simulink model "debugECDD"  (Simulink 7.2)
settings: Solver=ode1  StartTime=0.0  StopTime=50  FixedStep=0.002  RelTol=1e-3
values from neighbouring files (symbols this model uses):
  a = param.a    [DSC_Control_Analysis.m]    (also in DSC_Control_Analysis_Exp.m; DSC_Speed_Control_Analysis.m; EmpiricalTireCurves.m = 1.35; FFW_Fx.m = sqrt(curvature/(2*clothoidLength)))
  b = 1.15    [EmpiricalTireCurves.m]
  Cfls = Cfl    [EC_params_nissan.m]
  Crls = Crl    [EC_params_nissan.m]
  Iz = param.Iz    [DSC_Control_Analysis.m]    (also in DSC_Control_Analysis_Exp.m; DSC_Speed_Control_Analysis.m; EmpiricalTireCurves.m = 1300)
  K = 10    [EC_params_nissan.m]
  Ks = -10    [EC_params_nissan.m]
  Ksl = -10    [EC_params_nissan.m]
  Kt = 40000    [EC_params_nissan.m]
  Ku = -40000    [EC_params_nissan.m]
  m = 1724    [EmpiricalTireCurves.m]
  mu_s = mu_p    (= 0.6)    [EC_params_nissan.m]    (also in EmpiricalTireCurves.m = 0.55)
  Ns = 10    [EC_params_nissan.m]
  q = 1    [EC_params_nissan.m]
undefined symbols (not defined in the file or in its folder): c, Cfl, Crl, dden, denafilt, dnum, filtera, filterb, h_roll, Ifalphaparam, numafilt, param, rfl, rfr, rrl, rrr, sglu, slimFxl, slimFxu, sliml, slimMll, slimMlr, slimMul, slimMur, slimu, steering_limit, tw_m, wc
libraries: simulink x15, xpclib x3, UserBlocks x1
(part 2 of 3)

== system debugECDD/Envelope control with Differential drive/envelope controller with DD/control_on ==
  note: [Control on condition]
      | - Switch ON
      | - Brake OFF
      | - Vx > 2m/s
      | - GPS works
  Fault switch : Inport  OutDataType=sfix(16)  OutScaling=2^0
  brake_sw : Inport  Port=2  OutDataType=sfix(16)  OutScaling=2^0
  Vx : Inport  Port=3  OutDataType=sfix(16)  OutScaling=2^0
  Bus Selector1 : BusSelector  OutputSignals=signal2.Velocity Solution Status,signal1.Attitude Status
  Constant : Constant  Value=2  OutDataType=sfix(16)  OutScaling=2^0
  Constant1 : Constant  Value=3  OutDataType=sfix(16)  OutScaling=2^0
  Constant2 : Constant  Value=4  OutDataType=sfix(16)  OutScaling=2^0
  Data Type Conversion1 : DataTypeConversion  OutDataTypeMode=double  OutDataType=sfix(16)  OutScaling=2^0  OutDataTypeStr=double  RndMeth=Nearest  SaturateOnIntegerOverflow=on
  Data Type Conversion2 : DataTypeConversion  OutDataTypeMode=double  OutDataType=sfix(16)  OutScaling=2^0  OutDataTypeStr=double  RndMeth=Nearest  SaturateOnIntegerOverflow=on
  Data Type Conversion3 : DataTypeConversion  OutDataType=sfix(16)  OutScaling=2^0  RndMeth=Nearest  SaturateOnIntegerOverflow=on
  Logical Operator : Logic  Operator=NOT  AllPortsSameDT=off  OutDataTypeMode=boolean  OutDataTypeStr=boolean
  Logical Operator{1..4} (4 alike) : Logic  AllPortsSameDT=off  OutDataTypeMode=boolean  OutDataTypeStr=boolean
  Relational Operator : RelationalOperator  Operator=>  LogicOutDataTypeMode=boolean  OutDataTypeStr=boolean
  Relational Operator1 : RelationalOperator  Operator===  LogicOutDataTypeMode=boolean  OutDataTypeStr=boolean
  Relational Operator2 : RelationalOperator  Operator===  LogicOutDataTypeMode=boolean  OutDataTypeStr=boolean
  Rounding Function : Rounding  Operator=round
  Rounding Function1 : Rounding  Operator=round
  ON FLAG : Outport  OutDataType=sfix(16)  OutScaling=2^0
  tag scope: ECDDbrake=global, ECDDspeed=global, GPS_condition=global
  wires:
  Data Type Conversion3/1 -> [ECDDbrake], Logical Operator/1
  Logical Operator4/1 -> ON FLAG/1
  Logical Operator3/1 -> Logical Operator4/2, [GPS_condition]
  Logical Operator2/1 -> Logical Operator4/1
  Relational Operator2/1 -> Logical Operator3/2
  Relational Operator1/1 -> Logical Operator3/1
  Constant2/1 -> Relational Operator2/2
  Rounding Function1/1 -> Relational Operator2/1
  Constant1/1 -> Relational Operator1/1
  Rounding Function/1 -> Relational Operator1/2
  Data Type Conversion1/1 -> Rounding Function1/1
  Data Type Conversion2/1 -> Rounding Function/1
  [global_GPS] -> Bus Selector1/1
  Bus Selector1/2 -> Data Type Conversion1/1  "<Attitude Status>"
  Bus Selector1/1 -> Data Type Conversion2/1  "<Velocity Solution Status>"
  Relational Operator/1 -> [ECDDspeed], Logical Operator2/2
  Logical Operator1/1 -> Logical Operator2/1
  Constant/1 -> Relational Operator/2
  Vx/1 -> Relational Operator/1
  Logical Operator/1 -> Logical Operator1/2
  Fault switch/1 -> Logical Operator1/1
  brake_sw/1 -> Data Type Conversion3/1

== system debugECDD/Envelope control with Differential drive/envelope controller with DD/drive_dynamics ==
  In1 : Inport  OutDataType=sfix(16)  OutScaling=2^0
  Demux : Demux
  Discrete Transfer Fcn{,1..3} (4 alike) : DiscreteTransferFcn  Numerator=0.3297  Denominator=[1 -0.6703]  SampleTime=0.002
  Mux : Mux
  Out1 : Outport  OutDataType=sfix(16)  OutScaling=2^0
  wires:
  In1/1 -> Demux/1
  Mux/1 -> Out1/1
  Demux/1 -> Discrete Transfer Fcn/1
  Demux/2 -> Discrete Transfer Fcn1/1
  Demux/3 -> Discrete Transfer Fcn2/1
  Demux/4 -> Discrete Transfer Fcn3/1
  Discrete Transfer Fcn/1 -> Mux/1
  Discrete Transfer Fcn1/1 -> Mux/2
  Discrete Transfer Fcn2/1 -> Mux/3
  Discrete Transfer Fcn3/1 -> Mux/4

== system debugECDD/Envelope control with Differential drive/envelope controller with DD/reaction force control ==
  reaction 1 : Inport  OutDataType=sfix(16)  OutScaling=2^0
  reaction 2 : Inport  Port=2  OutDataType=sfix(16)  OutScaling=2^0
  Constant : Constant  Value=0  OutDataType=sfix(16)  OutScaling=2^0
  Constant1 : Constant  Value=0  OutDataType=sfix(16)  OutScaling=2^0
  Constant2 : Constant  Value=0  OutDataType=sfix(16)  OutScaling=2^0
  Terminator : Terminator
  Terminator1 : Terminator
  steer force : Outport  OutDataType=sfix(16)  OutScaling=2^0
  ACC pedal force : Outport  Port=2  OutDataType=sfix(16)  OutScaling=2^0
  Brake pedal force1 : Outport  Port=3  OutDataType=sfix(16)  OutScaling=2^0
  wires:
  reaction 2/1 -> Terminator1/1
  reaction 1/1 -> Terminator/1
  Constant2/1 -> Brake pedal force1/1
  Constant1/1 -> ACC pedal force/1
  Constant/1 -> steer force/1

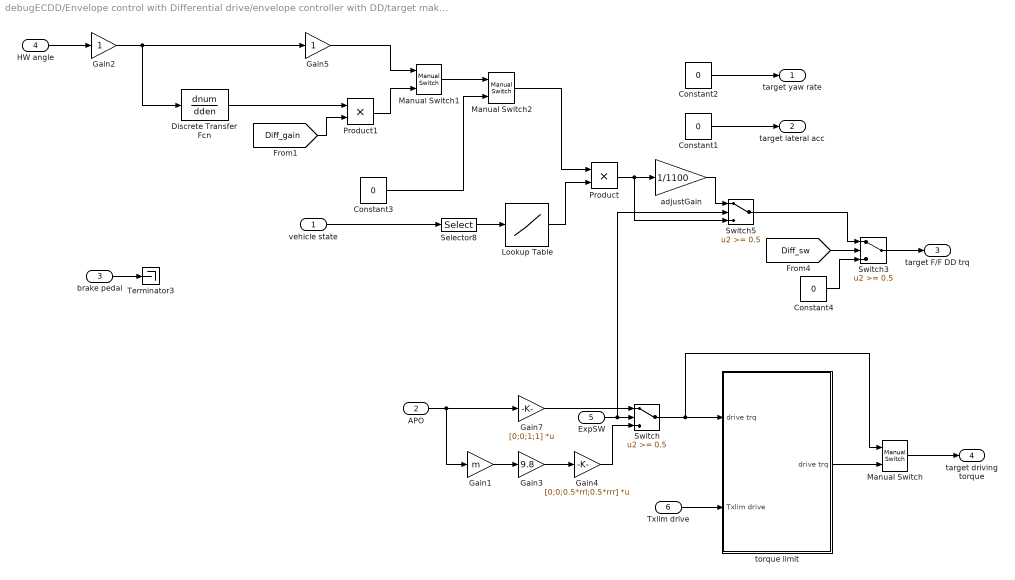
== system debugECDD/Envelope control with Differential drive/envelope controller with DD/target making ==
  vehicle state : Inport  OutDataType=sfix(16)  OutScaling=2^0
  APO : Inport  Port=2  OutDataType=sfix(16)  OutScaling=2^0
  brake pedal : Inport  Port=3  OutDataType=sfix(16)  OutScaling=2^0
  HW angle : Inport  Port=4  OutDataType=sfix(16)  OutScaling=2^0
  ExpSW : Inport  Port=5  OutDataType=sfix(16)  OutScaling=2^0
  Txlim drive : Inport  Port=6  OutDataType=sfix(16)  OutScaling=2^0
  Constant{1..4} (4 alike) : Constant  Value=0  OutDataType=sfix(16)  OutScaling=2^0
  Discrete Transfer Fcn : DiscreteTransferFcn  Numerator=dnum  Denominator=dden  SampleTime=0.002
  Gain1 : Gain  Gain=m  ParameterDataType=sfix(16)  ParameterScaling=2^0  OutDataType=sfix(16)  OutScaling=2^0
  Gain2 : Gain  ParameterDataType=sfix(16)  ParameterScaling=2^0  OutDataType=sfix(16)  OutScaling=2^0
  Gain3 : Gain  Gain=9.8  ParameterDataType=sfix(16)  ParameterScaling=2^0  OutDataType=sfix(16)  OutScaling=2^0
  Gain4 : Gain  Gain=[0;0;0.5*rrl;0.5*rrr]  Multiplication=Matrix(K*u)  ParameterDataType=sfix(16)  ParameterScaling=2^0  OutDataType=sfix(16)  OutScaling=2^0
  Gain5 : Gain  ParameterDataType=sfix(16)  ParameterScaling=2^0  OutDataType=sfix(16)  OutScaling=2^0
  Gain7 : Gain  Gain=[0;0;1;1]  Multiplication=Matrix(K*u)  ParameterDataType=sfix(16)  ParameterScaling=2^0  OutDataType=sfix(16)  OutScaling=2^0
  Lookup Table : Lookup  InputValues=[0;1;2;3]  Table=[0;0;1;1]  OutDataType=sfix(16)  OutScaling=2^0
  Manual Switch : simulink/Signal Routing/Manual Switch  SystemSampleTime=-1  sw=0  action=0  varsize=off
  Manual Switch1 : simulink/Signal Routing/Manual Switch  SystemSampleTime=-1  sw=0  action=0  varsize=off
  Manual Switch2 : simulink/Signal Routing/Manual Switch  SystemSampleTime=-1  sw=1  action=0  varsize=off
  Product : Product  OutDataType=sfix(16)  OutScaling=2^0  RndMeth=Zero
  Product1 : Product  OutDataType=sfix(16)  OutScaling=2^0  RndMeth=Zero
  Selector8 : Selector  InputPortWidth=12  IndexOptions=Index vector (dialog)  Indices=5  OutputSizes=1
  Switch : Switch  Threshold=0.5  OutDataType=sfix(16)  OutScaling=2^0
  Switch3 : Switch  Threshold=0.5
  Switch5 : Switch  Threshold=0.5
  Terminator3 : Terminator
  adjustGain : Gain  Gain=1/1100  ParameterDataType=sfix(16)  ParameterScaling=2^0  OutDataType=sfix(16)  OutScaling=2^0
  torque limit : Subsystem
  target yaw rate : Outport  OutDataType=sfix(16)  OutScaling=2^0
  target lateral acc : Outport  Port=2  OutDataType=sfix(16)  OutScaling=2^0
  target F/F DD trq : Outport  Port=3  OutDataType=sfix(16)  OutScaling=2^0
  target driving torque : Outport  Port=4  OutDataType=sfix(16)  OutScaling=2^0
  wires:
  Gain3/1 -> Gain4/1
  Gain1/1 -> Gain3/1
  Constant1/1 -> target lateral acc/1
  brake pedal/1 -> Terminator3/1
  ExpSW/1 -> Switch/2, Switch5/2
  Gain4/1 -> Switch/3
  APO/1 -> Gain1/1, Gain7/1
  Gain7/1 -> Switch/1
  Switch/1 -> torque limit/1("drive trq "), Manual Switch/1
  Txlim drive/1 -> torque limit/2(Txlim drive)
  torque limit/1(drive trq) -> Manual Switch/2
  Manual Switch/1 -> target driving torque/1
  Constant2/1 -> target yaw rate/1
  HW angle/1 -> Gain2/1
  Gain2/1 -> Gain5/1, Discrete Transfer Fcn/1
  vehicle state/1 -> Selector8/1
  Selector8/1 -> Lookup Table/1
  Lookup Table/1 -> Product/2
  Product1/1 -> Manual Switch1/2
  Gain5/1 -> Manual Switch1/1
  Manual Switch2/1 -> Product/1
  Manual Switch1/1 -> Manual Switch2/1
  Constant3/1 -> Manual Switch2/2
  [Diff_sw] -> Switch3/2
  Constant4/1 -> Switch3/3
  Switch3/1 -> target F/F DD trq/1
  Discrete Transfer Fcn/1 -> Product1/1
  [Diff_gain] -> Product1/2
  adjustGain/1 -> Switch5/1
  Product/1 -> adjustGain/1, Switch5/3
  Switch5/1 -> Switch3/1

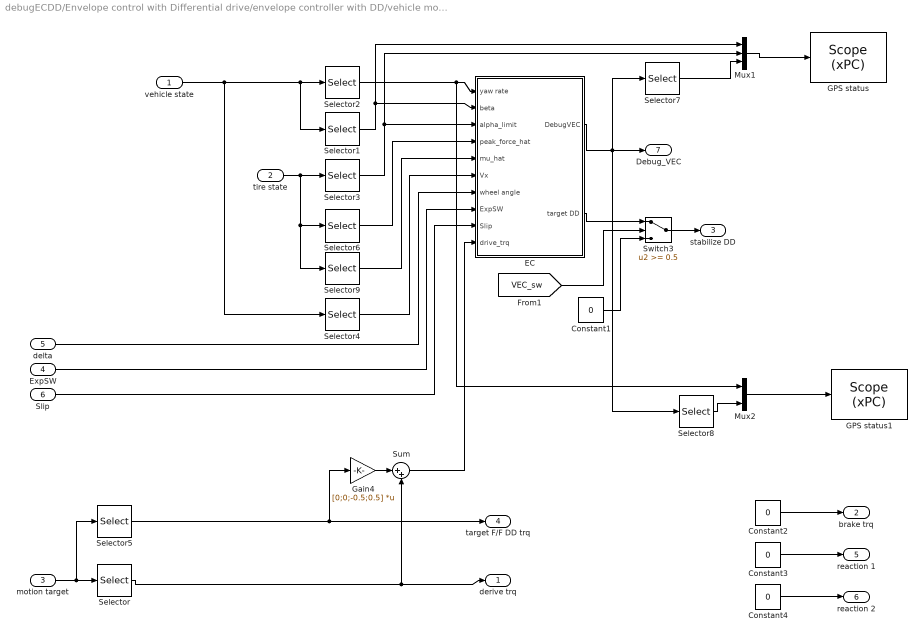
== system debugECDD/Envelope control with Differential drive/envelope controller with DD/vehicle motion control ==
  vehicle state : Inport  OutDataType=sfix(16)  OutScaling=2^0
  tire state : Inport  Port=2  OutDataType=sfix(16)  OutScaling=2^0
  motion target : Inport  Port=3  OutDataType=sfix(16)  OutScaling=2^0
  ExpSW : Inport  Port=4  OutDataType=sfix(16)  OutScaling=2^0
  delta : Inport  Port=5  OutDataType=sfix(16)  OutScaling=2^0
  Slip : Inport  Port=6  OutDataType=sfix(16)  OutScaling=2^0
  Constant{1..4} (4 alike) : Constant  Value=0  OutDataType=sfix(16)  OutScaling=2^0
  EC : Subsystem
  GPS status : xpclib/Misc./Scope (xPC)   SystemSampleTime=-1  scopeno=1  scopetype=Target  autostart=on  viewmode=Graphical sliding  formatstr='%15.6f'  grid=on  ylimits=[-1,1]  nosamples=round(1/Ts)  noprepostsamples=0  interleave=1  triggermode=FreeRun  triggersignal=1  triggerlevel=0.0  triggerslope=Either  triggerscope=1  triggersample=0  filename=data.dat  mode=Lazy  writesize=512  autorestart=off
  GPS status1 : xpclib/Misc./Scope (xPC)   SystemSampleTime=-1  scopeno=4  scopetype=Target  autostart=on  viewmode=Graphical sliding  formatstr='%15.6f'  grid=on  ylimits=[-1,1]  nosamples=round(1/Ts)  noprepostsamples=0  interleave=1  triggermode=FreeRun  triggersignal=1  triggerlevel=0.0  triggerslope=Either  triggerscope=1  triggersample=0  filename=data.dat  mode=Lazy  writesize=512  autorestart=off
  Gain4 : Gain  Gain=[0;0;-0.5;0.5]  Multiplication=Matrix(K*u)  ParameterDataType=sfix(16)  ParameterScaling=2^0  OutDataType=sfix(16)  OutScaling=2^0
  Mux1 : Mux  Inputs=3
  Mux2 : Mux  Inputs=2
  Selector : Selector  InputPortWidth=7  IndexOptions=Index vector (dialog)  Indices=[4:7]  OutputSizes=1
  Selector1 : Selector  InputPortWidth=12  IndexOptions=Index vector (dialog)  Indices=12  OutputSizes=1
  Selector2 : Selector  InputPortWidth=12  IndexOptions=Index vector (dialog)  Indices=7  OutputSizes=1
  Selector3 : Selector  InputPortWidth=9  IndexOptions=Index vector (dialog)  Indices=[7:8]  OutputSizes=1
  Selector4 : Selector  InputPortWidth=12  IndexOptions=Index vector (dialog)  Indices=5  OutputSizes=1
  Selector5 : Selector  InputPortWidth=7  IndexOptions=Index vector (dialog)  Indices=3  OutputSizes=1
  Selector6 : Selector  InputPortWidth=9  IndexOptions=Index vector (dialog)  Indices=[3:6]  OutputSizes=1
  Selector7 : Selector  InputPortWidth=11  IndexOptions=Index vector (dialog)  Indices=[8 9]  OutputSizes=1
  Selector8 : Selector  InputPortWidth=11  IndexOptions=Index vector (dialog)  Indices=[6 7]  OutputSizes=1
  Selector9 : Selector  InputPortWidth=9  IndexOptions=Index vector (dialog)  Indices=9  OutputSizes=1
  Sum : Sum  Inputs=|++  OutDataType=sfix(16)  OutScaling=2^0
  Switch3 : Switch  Threshold=0.5
  derive trq : Outport  OutDataType=sfix(16)  OutScaling=2^0
  brake trq : Outport  Port=2  OutDataType=sfix(16)  OutScaling=2^0
  stabilize DD : Outport  Port=3  OutDataType=sfix(16)  OutScaling=2^0
  target F/F DD trq : Outport  Port=4  OutDataType=sfix(16)  OutScaling=2^0
  reaction 1 : Outport  Port=5  OutDataType=sfix(16)  OutScaling=2^0
  reaction 2 : Outport  Port=6  OutDataType=sfix(16)  OutScaling=2^0
  Debug_VEC : Outport  Port=7  OutDataType=sfix(16)  OutScaling=2^0
  wires:
  Mux1/1 -> GPS status/1
  Selector7/1 -> Mux1/3
  EC/1(DebugVEC) -> Selector7/1, Debug_VEC/1, Selector8/1
  Selector4/1 -> EC/6(Vx)
  Constant1/1 -> Switch3/3
  EC/2(target DD) -> Switch3/1
  [VEC_sw] -> Switch3/2
  delta/1 -> EC/7(wheel angle)
  tire state/1 -> Selector3/1, Selector6/1, Selector9/1
  Selector3/1 -> EC/3(alpha_limit), Mux1/2
  Selector1/1 -> Mux1/1, EC/2(beta)
  vehicle state/1 -> Selector1/1, Selector2/1, Selector4/1
  Selector2/1 -> EC/1(yaw rate), Mux2/1
  motion target/1 -> Selector/1, Selector5/1
  Constant4/1 -> reaction 2/1
  Constant3/1 -> reaction 1/1
  Constant2/1 -> brake trq/1
  Mux2/1 -> GPS status1/1
  Selector8/1 -> Mux2/2
  Selector6/1 -> EC/4(peak_force_hat)
  ExpSW/1 -> EC/8(ExpSW)
  Slip/1 -> EC/9(Slip)
  Switch3/1 -> stabilize DD/1
  Selector9/1 -> EC/5(mu_hat)
  Selector/1 -> derive trq/1, Sum/2
  Selector5/1 -> target F/F DD trq/1, Gain4/1
  Gain4/1 -> Sum/1
  Sum/1 -> EC/10(drive_trq)

== system debugECDD/Envelope control with Differential drive/envelope controller with DD/Control switch/Delay ==
  In1 : Inport  OutDataType=sfix(16)  OutScaling=2^0
  Unit Delay{,1..4} (5 alike) : UnitDelay  X0=2  SampleTime=0.002
  Out1 : Outport  OutDataType=sfix(16)  OutScaling=2^0
  wires:
  In1/1 -> Unit Delay/1
  Unit Delay/1 -> Unit Delay1/1
  Unit Delay1/1 -> Unit Delay2/1
  Unit Delay2/1 -> Unit Delay3/1
  Unit Delay3/1 -> Unit Delay4/1
  Unit Delay4/1 -> Out1/1

== system debugECDD/Envelope control with Differential drive/envelope controller with DD/Control switch/Triggered Subsystem1 ==
  In1 : Inport  OutDataType=sfix(16)  OutScaling=2^0
  Trigger : TriggerPort
  Constant : Constant  OutDataType=sfix(16)  OutScaling=2^0
  Constant1 : Constant  OutDataType=sfix(16)  OutScaling=2^0
  Sum : Sum  Inputs=|++  OutDataType=sfix(16)  OutScaling=2^0
  Switch : Switch  Threshold=4.5  OutDataType=sfix(16)  OutScaling=2^0
  Out1 : Outport  OutDataType=sfix(16)  OutScaling=2^0  InitialOutput=2
  wires:
  In1/1 -> Sum/1
  Constant/1 -> Sum/2
  Sum/1 -> Switch/2, Switch/3
  Constant1/1 -> Switch/1
  Switch/1 -> Out1/1

== system debugECDD/Envelope control with Differential drive/envelope controller with DD/Tire force control/limit_cal ==
  muFz : Inport  OutDataType=sfix(16)  OutScaling=2^0
  alpha : Inport  Port=2  OutDataType=sfix(16)  OutScaling=2^0
  ExpSW : Inport  Port=3  OutDataType=sfix(16)  OutScaling=2^0
  stabilize DD : Inport  Port=4  OutDataType=sfix(16)  OutScaling=2^0
  Fx_limit_cal : Subsystem
  Fx_limit_cal1 : Subsystem
  MinMax{1..4} (4 alike) : MinMax  Inputs=2  OutDataType=sfix(16)  OutScaling=2^0
  Mux1 : Mux
  Mux7 : Mux
  RL & RR max : Constant  Value=3  OutDataType=sfix(16)  OutScaling=2^0
  RL & RR max1 : Constant  Value=3  OutDataType=sfix(16)  OutScaling=2^0
  RL min : Constant  Value=0.75  OutDataType=sfix(16)  OutScaling=2^0
  RL min1 : Constant  Value=0.75  OutDataType=sfix(16)  OutScaling=2^0
  RR min : Constant  Value=0.75  OutDataType=sfix(16)  OutScaling=2^0
  RR min1 : Constant  Value=0.75  OutDataType=sfix(16)  OutScaling=2^0
  Selector1 : Selector  InputPortWidth=4  IndexOptions=Index vector (dialog)  Indices=3  OutputSizes=1
  Selector2 : Selector  InputPortWidth=4  IndexOptions=Index vector (dialog)  Indices=3  OutputSizes=1
  Selector3 : Selector  InputPortWidth=4  IndexOptions=Index vector (dialog)  Indices=1  OutputSizes=1
  Selector8 : Selector  InputPortWidth=4  IndexOptions=Index vector (dialog)  Indices=1  OutputSizes=1
  Sum : Sum  Inputs=|++  OutDataType=sfix(16)  OutScaling=2^0
  Sum1 : Sum  Inputs=|++  OutDataType=sfix(16)  OutScaling=2^0
  Switch1 : Switch  Threshold=0.5
  Switch4 : Switch  Threshold=0.5
  adjustGain : Gain  Gain=1/1100  ParameterDataType=sfix(16)  ParameterScaling=2^0  OutDataType=sfix(16)  OutScaling=2^0
  adjustGain1 : Gain  Gain=1/1100  ParameterDataType=sfix(16)  ParameterScaling=2^0  OutDataType=sfix(16)  OutScaling=2^0
  pedal offset : Constant  Value=1.75  OutDataType=sfix(16)  OutScaling=2^0
  pedal offset1 : Constant  Value=1.75  OutDataType=sfix(16)  OutScaling=2^0
  slip_limit_cal1 : Subsystem
  slim : Outport  OutDataType=sfix(16)  OutScaling=2^0
  Txlim : Outport  Port=2  OutDataType=sfix(16)  OutScaling=2^0
  Txlim drive : Outport  Port=3  OutDataType=sfix(16)  OutScaling=2^0
  wires:
  Switch4/1 -> Txlim/1
  Fx_limit_cal/1(Txlim) -> Switch4/3, adjustGain/1
  ExpSW/1 -> Switch4/2, Switch1/2
  slip_limit_cal1/1(slim) -> Fx_limit_cal/2(slim), slim/1
  muFz/1 -> slip_limit_cal1/3(muFz), Fx_limit_cal/3(muFz), Fx_limit_cal1/3(muFz)
  alpha/1 -> slip_limit_cal1/1(alpha), Fx_limit_cal/1(alpha), Fx_limit_cal1/1(alpha)
  Selector8/1 -> MinMax4/1
  Selector1/1 -> MinMax1/1
  RL & RR max/1 -> MinMax4/2, MinMax1/2
  MinMax4/1 -> Mux7/1
  RL min/1 -> Mux7/2
  MinMax1/1 -> Mux7/3
  RR min/1 -> Mux7/4
  Mux7/1 -> Switch4/1
  Sum/1 -> Selector8/1, Selector1/1
  adjustGain/1 -> Sum/1
  pedal offset/1 -> Sum/2
  stabilize DD/1 -> slip_limit_cal1/2(stabilize DD), Fx_limit_cal/4(stabilize DD)
  Switch1/1 -> Txlim drive/1
  Fx_limit_cal1/1(Txlim drive) -> adjustGain1/1, Switch1/3, Fx_limit_cal/5(Txlim drive)
  Selector3/1 -> MinMax3/1
  Selector2/1 -> MinMax2/1
  RL & RR max1/1 -> MinMax2/2, MinMax3/2
  MinMax3/1 -> Mux1/1
  RL min1/1 -> Mux1/2
  MinMax2/1 -> Mux1/3
  RR min1/1 -> Mux1/4
  Mux1/1 -> Switch1/1
  Sum1/1 -> Selector2/1, Selector3/1
  adjustGain1/1 -> Sum1/1
  pedal offset1/1 -> Sum1/2
  slip_limit_cal1/2(slim drive) -> Fx_limit_cal1/2(slim drive)

== system debugECDD/Envelope control with Differential drive/envelope controller with DD/Tire force control/s_cal  ==
  note: Vx
  Omega : Inport  OutDataType=sfix(16)  OutScaling=2^0
  Vx : Inport  Port=2  OutDataType=sfix(16)  OutScaling=2^0
  yaw rate : Inport  Port=3  OutDataType=sfix(16)  OutScaling=2^0
  ExpSW : Inport  Port=4  OutDataType=sfix(16)  OutScaling=2^0
  Add4 : Sum  Inputs=+-  OutDataType=sfix(16)  OutScaling=2^-10
  Add5 : Sum  Inputs=+-  OutDataType=sfix(16)  OutScaling=2^-10
  Butterworth Filter : DiscreteFilter  Numerator=filterb  Denominator=filtera  SampleTime=0.002
  Butterworth Filter1 : DiscreteFilter  Numerator=filterb  Denominator=filtera  SampleTime=0.002
  Demux4 : Demux
  Divide : Product  Inputs=*/  OutDataType=sfix(16)  OutScaling=2^-10
  Divide1 : Product  Inputs=*/  OutDataType=sfix(16)  OutScaling=2^-10
  Gain1 : Gain  Gain=rrl  ParameterDataType=sfix(16)  ParameterScaling=2^0  OutDataType=sfix(16)  OutScaling=2^0
  Gain2 : Gain  Gain=rrr  ParameterDataType=sfix(16)  ParameterScaling=2^0  OutDataType=sfix(16)  OutScaling=2^0
  Gain3 : Gain  Gain=c  ParameterDataType=sfix(16)  ParameterScaling=2^0  OutDataType=sfix(16)  OutScaling=2^0
  Manual Switch : simulink/Signal Routing/Manual Switch  SystemSampleTime=-1  sw=0  action=0  varsize=off
  Manual Switch1 : simulink/Signal Routing/Manual Switch  SystemSampleTime=-1  sw=0  action=0  varsize=off
  Mux : Mux  Inputs=2
  Product : Product  OutDataType=sfix(16)  OutScaling=2^0  RndMeth=Zero
  Relational Operator : RelationalOperator  Operator=<  LogicOutDataTypeMode=boolean  OutDataTypeStr=boolean
  Relational Operator1 : RelationalOperator  Operator=<  LogicOutDataTypeMode=boolean  OutDataTypeStr=boolean
  Saturation : Saturate  UpperLimit=0.99  LowerLimit=-0.99
  Saturation1 : Saturate  UpperLimit=0.99  LowerLimit=-0.99
  Sum : Sum  Inputs=|+-  OutDataType=sfix(16)  OutScaling=2^0
  Sum1 : Sum  Inputs=++|  OutDataType=sfix(16)  OutScaling=2^0
  Switch : Switch  Threshold=0.5
  Switch1 : Switch  Threshold=0.5
  Terminator1 : Terminator
  Terminator2 : Terminator
  prevent zero : Subsystem
  prevent zero1 : Subsystem
  s : Outport  OutDataType=sfix(16)  OutScaling=2^0
  wires:
  Manual Switch1/1 -> Sum1/2, Sum/1
  Gain2/1 -> Relational Operator/2, Add5/2, Switch/1
  Gain1/1 -> Relational Operator1/2, Add4/2, Switch1/1
  Gain3/1 -> Sum1/1, Sum/2
  Sum1/1 -> Relational Operator/1, Add5/1, Switch/3
  Sum/1 -> Relational Operator1/1, Add4/1, Switch1/3
  Product/1 -> Gain3/1
  ExpSW/1 -> Product/2
  yaw rate/1 -> Butterworth Filter1/1, Manual Switch/1
  Demux4/2 -> Terminator1/1
  Demux4/1 -> Terminator2/1
  Mux/1 -> s/1
  Divide1/1 -> Saturation/1
  Divide/1 -> Saturation1/1
  Omega/1 -> Demux4/1
  Add5/1 -> Divide1/1
  Add4/1 -> Divide/1
  Demux4/4 -> Gain2/1
  Demux4/3 -> Gain1/1
  Vx/1 -> Butterworth Filter/1, Manual Switch1/1
  prevent zero/1(Out1) -> Divide/2
  prevent zero1/1(Out1) -> Divide1/2
  Switch/1 -> prevent zero1/1(In1)
  Relational Operator/1 -> Switch/2
  Switch1/1 -> prevent zero/1(In1)
  Relational Operator1/1 -> Switch1/2
  Saturation/1 -> Mux/2
  Saturation1/1 -> Mux/1
  Manual Switch/1 -> Product/1
  Butterworth Filter1/1 -> Manual Switch/2
  Butterworth Filter/1 -> Manual Switch1/2

== system debugECDD/Envelope control with Differential drive/envelope controller with DD/Tire force control/slip_limit ==
  s : Inport  OutDataType=sfix(16)  OutScaling=2^0
  slim : Inport  Port=2  OutDataType=sfix(16)  OutScaling=2^0
  Constant4 : Constant  Value=[0;0]  OutDataType=sfix(16)  OutScaling=2^0
  Data Type Conversion : DataTypeConversion  OutDataType=sfix(16)  OutScaling=2^0
  Data Type Conversion1 : DataTypeConversion  OutDataType=sfix(16)  OutScaling=2^0
  Demux2 : Demux  Outputs=2
  Demux3 : Demux  Outputs=2
  Demux4 : Demux  Outputs=2
  Demux5 : Demux  Outputs=3
  Demux6 : Demux  Outputs=3
  Gain : Gain  Gain=[1 0 0 0;0 1 0 0;0 0 1 1;0 0 1 1]  Multiplication=Matrix(K*u)  ParameterDataType=sfix(16)  ParameterScaling=2^0  OutDataType=sfix(16)  OutScaling=2^0
  Manual Switch : simulink/Signal Routing/Manual Switch  SystemSampleTime=-1  sw=0  action=0  varsize=off
  Mux1 : Mux  Inputs=5
  Mux2 : Mux  Inputs=5
  Mux3 : Mux  Inputs=2
  Mux8 : Mux  Inputs=3
  S-Function : S-Function  FunctionName=TECslipcont  Parameters=[Ksl, Kt]  EnableBusSupport=off
  S-Function1 : S-Function  FunctionName=TECslipcont  Parameters=[Ksl, Kt]  EnableBusSupport=off
  Selector1 : Selector  InputPortWidth=4  IndexOptions=Index vector (dialog)  Indices=[2,1]  OutputSizes=1
  Selector3 : Selector  InputPortWidth=4  IndexOptions=Index vector (dialog)  Indices=[4 3]  OutputSizes=1
  Selector4 : Selector  InputPortWidth=3  IndexOptions=Index vector (dialog)  Indices=3  OutputSizes=1
  Selector5 : Selector  InputPortWidth=3  IndexOptions=Index vector (dialog)  Indices=3  OutputSizes=1
  Switch2 : Switch  Threshold=0.5
  Terminator1 : Terminator
  Terminator2 : Terminator
  Unit Delay : UnitDelay  Orientation=left  SampleTime=0.002
  Unit Delay1 : UnitDelay  Orientation=left  SampleTime=0.002
  Zero-Order Hold : ZeroOrderHold  SampleTime=0.002
  Zero-Order Hold1 : ZeroOrderHold  SampleTime=0.002
  DebugTEC : Outport  OutDataType=sfix(16)  OutScaling=2^0
  drive trq : Outport  Port=2  OutDataType=sfix(16)  OutScaling=2^0
  wires:
  Data Type Conversion1/1 -> Mux2/4
  Data Type Conversion/1 -> Mux1/4
  [sliplimit_sw] -> Data Type Conversion1/1
  Unit Delay1/1 -> Mux2/5
  [sliplimit_sw] -> Data Type Conversion/1
  Unit Delay/1 -> Mux1/5
  Selector5/1 -> Mux3/2
  Selector4/1 -> Mux3/1
  Mux3/1 -> DebugTEC/1
  Demux6/3 -> Terminator1/1
  Demux5/3 -> Terminator2/1
  Demux4/2 -> Mux2/3
  Demux4/1 -> Mux2/2
  Demux3/2 -> Mux1/3
  Demux3/1 -> Mux1/2
  Demux6/1 -> Mux8/3
  Demux5/1 -> Mux8/2
  Demux6/2 -> Unit Delay1/1
  S-Function1/1 -> Selector5/1, Demux6/1
  Mux2/1 -> S-Function1/1
  Demux5/2 -> Unit Delay/1
  S-Function/1 -> Selector4/1, Demux5/1
  Mux1/1 -> S-Function/1
  s/1 -> Demux2/1
  Constant4/1 -> Mux8/1
  Selector1/1 -> Zero-Order Hold/1
  Demux2/1 -> Mux1/1
  Demux2/2 -> Mux2/1
  slim/1 -> Selector1/1, Selector3/1
  Zero-Order Hold/1 -> Demux3/1
  Zero-Order Hold1/1 -> Demux4/1
  Selector3/1 -> Zero-Order Hold1/1
  [TEC_sw] -> Switch2/2
  Mux8/1 -> Switch2/1, Gain/1, Manual Switch/2
  Gain/1 -> Manual Switch/1
  Manual Switch/1 -> Switch2/3
  Switch2/1 -> drive trq/1

== system debugECDD/Envelope control with Differential drive/envelope controller with DD/Tire force control/steering control ==
  yaw rate : Inport  OutDataType=sfix(16)  OutScaling=2^0
  beta : Inport  Port=2  OutDataType=sfix(16)  OutScaling=2^0
  Vx : Inport  Port=3  OutDataType=sfix(16)  OutScaling=2^0
  alphalimit : Inport  Port=4  OutDataType=sfix(16)  OutScaling=2^0
  wheel angle : Inport  Port=5  OutDataType=sfix(16)  OutScaling=2^0
  Demux1 : Demux  Outputs=2
  MinMax2 : MinMax  OutDataType=sfix(16)  OutScaling=2^0
  MinMax3 : MinMax  Function=max  OutDataType=sfix(16)  OutScaling=2^0
  Mux3 : Mux  Inputs=2
  Mux4 : Mux  Inputs=2
  Mux5 : Mux  Inputs=2
  Selector : Selector  InputPortWidth=2  IndexOptions=Index vector (dialog)  Indices=1  OutputSizes=1
  Zero-Order Hold4 : ZeroOrderHold  SampleTime=0.002
  delta limit cal : Subsystem
  wheel angle1 : Outport  OutDataType=sfix(16)  OutScaling=2^0
  wires:
  Selector/1 -> delta limit cal/4(aflim)
  alphalimit/1 -> Selector/1
  yaw rate/1 -> delta limit cal/3(yaw rate)
  beta/1 -> delta limit cal/2(beta)
  delta limit cal/1(upper lim) -> Mux3/1
  delta limit cal/2(lower lim) -> Mux3/2
  wheel angle/1 -> Zero-Order Hold4/1
  Mux4/1 -> MinMax2/1
  MinMax2/1 -> Mux5/1
  Mux5/1 -> MinMax3/1
  Demux1/1 -> Mux4/2
  Demux1/2 -> Mux5/2
  Mux3/1 -> Demux1/1
  MinMax3/1 -> wheel angle1/1
  Zero-Order Hold4/1 -> Mux4/1
  Vx/1 -> delta limit cal/1(Vx)

== system debugECDD/Envelope control with Differential drive/envelope controller with DD/Tire force control/torque limit ==
  "drive trq " : Inport  OutDataType=sfix(16)  OutScaling=2^0
  Txlim : Inport  Port=2  OutDataType=sfix(16)  OutScaling=2^0
  MinMax4 : MinMax  Inputs=2  OutDataType=sfix(16)  OutScaling=2^0
  MinMax5 : MinMax  Function=max  Inputs=2  OutDataType=sfix(16)  OutScaling=2^0
  MinMax6 : MinMax  Inputs=2  OutDataType=sfix(16)  OutScaling=2^0
  MinMax7 : MinMax  Function=max  Inputs=2  OutDataType=sfix(16)  OutScaling=2^0
  Mux1 : Mux  Inputs=3
  Selector1 : Selector  InputPortWidth=4  IndexOptions=Index vector (dialog)  Indices=[1 2]  OutputSizes=1
  Selector10 : Selector  InputPortWidth=4  IndexOptions=Index vector (dialog)  Indices=1  OutputSizes=1
  Selector11 : Selector  InputPortWidth=4  IndexOptions=Index vector (dialog)  Indices=3  OutputSizes=1
  Selector12 : Selector  InputPortWidth=4  IndexOptions=Index vector (dialog)  Indices=2  OutputSizes=1
  Selector13 : Selector  InputPortWidth=4  IndexOptions=Index vector (dialog)  Indices=4  OutputSizes=1
  Selector8 : Selector  InputPortWidth=4  IndexOptions=Index vector (dialog)  Indices=3  OutputSizes=1
  Selector9 : Selector  InputPortWidth=4  IndexOptions=Index vector (dialog)  Indices=4  OutputSizes=1
  drive trq : Outport  OutDataType=sfix(16)  OutScaling=2^0
  wires:
  Selector8/1 -> MinMax4/1
  Selector10/1 -> MinMax4/2
  MinMax4/1 -> MinMax5/1
  Selector12/1 -> MinMax5/2
  Selector9/1 -> MinMax6/1
  Selector11/1 -> MinMax6/2
  MinMax6/1 -> MinMax7/1
  Selector13/1 -> MinMax7/2
  MinMax5/1 -> Mux1/2
  MinMax7/1 -> Mux1/3
  Mux1/1 -> drive trq/1
  "drive trq "/1 -> Selector9/1, Selector8/1, Selector1/1
  Txlim/1 -> Selector10/1, Selector12/1, Selector13/1, Selector11/1
  Selector1/1 -> Mux1/1

== system debugECDD/Envelope control with Differential drive/envelope controller with DD/Tire state estimation/Load Transfer ==
  Fx : Inport  OutDataType=sfix(16)  OutScaling=2^0
  Fy : Inport  Port=2  OutDataType=sfix(16)  OutScaling=2^0
  Fz_fl : Fcn  Expr=(b*m*9.8-h_roll*u[1])*(tw_m/2*m*9.8-h_roll*u[2])/((a+b)*2*tw_m/2*m*9.8)
  Fz_fr : Fcn  Expr=(b*m*9.8-h_roll*u[1])*(tw_m/2*m*9.8+h_roll*u[2])/((a+b)*2*tw_m/2*m*9.8)
  Fz_rl : Fcn  Expr=(a*m*9.8+h_roll*u[1])*(tw_m/2*m*9.8-h_roll*u[2])/((a+b)*2*tw_m/2*m*9.8)
  Fz_rr : Fcn  Expr=(a*m*9.8+h_roll*u[1])*(tw_m/2*m*9.8+h_roll*u[2])/((a+b)*2*tw_m/2*m*9.8)
  Mux : Mux  Inputs=2
  Mux1 : Mux
  Fz : Outport  OutDataType=sfix(16)  OutScaling=2^0
  wires:
  Fy/1 -> Mux/2
  Mux/1 -> Fz_fl/1, Fz_rr/1, Fz_rl/1, Fz_fr/1
  Fz_fl/1 -> Mux1/1
  Fz_fr/1 -> Mux1/2
  Fz_rl/1 -> Mux1/3
  Fz_rr/1 -> Mux1/4
  Mux1/1 -> Fz/1
  Fx/1 -> Mux/1

== system debugECDD/Envelope control with Differential drive/envelope controller with DD/Tire state estimation/Tire slip angle ==
  delta : Inport  OutDataType=sfix(16)  OutScaling=2^0
  beta : Inport  Port=2  OutDataType=sfix(16)  OutScaling=2^0
  r : Inport  Port=3  OutDataType=sfix(16)  OutScaling=2^0
  Vx : Inport  Port=4  OutDataType=sfix(16)  OutScaling=2^0
  Add : Sum  Inputs=++-  OutDataType=sfix(16)  OutScaling=2^-10
  Add1 : Sum  Inputs=-+  OutDataType=sfix(16)  OutScaling=2^-10
  Constant : Constant  Value=a  OutDataType=sfix(16)  OutScaling=2^0
  Constant1 : Constant  Value=b  OutDataType=sfix(16)  OutScaling=2^0
  Divide : Product  Inputs=**/  OutDataType=sfix(16)  OutScaling=2^-10
  Divide1 : Product  Inputs=**/  OutDataType=sfix(16)  OutScaling=2^-10
  af : Outport  OutDataType=sfix(16)  OutScaling=2^0
  ar : Outport  Port=2  OutDataType=sfix(16)  OutScaling=2^0
  wires:
  Constant/1 -> Divide/1
  Divide/1 -> Add/1
  r/1 -> Divide/2, Divide1/2
  beta/1 -> Add/2, Add1/2
  Vx/1 -> Divide/3, Divide1/3
  delta/1 -> Add/3
  Add/1 -> af/1
  Constant1/1 -> Divide1/1
  Divide1/1 -> Add1/1
  Add1/1 -> ar/1

== system debugECDD/Envelope control with Differential drive/envelope controller with DD/Tire state estimation/alpha_limit_cal ==
  muFz : Inport  OutDataType=sfix(16)  OutScaling=2^0
  Gain : Gain  Gain=3/Cfls  ParameterDataType=sfix(16)  ParameterScaling=2^0  OutDataType=sfix(16)  OutScaling=2^0
  Gain1 : Gain  Gain=3/Crls  ParameterDataType=sfix(16)  ParameterScaling=2^0  OutDataType=sfix(16)  OutScaling=2^0
  MinMax : MinMax  Function=max  OutDataType=sfix(16)  OutScaling=2^0
  MinMax1 : MinMax  Function=max  OutDataType=sfix(16)  OutScaling=2^0
  Mux : Mux  Inputs=2
  Selector : Selector  InputPortWidth=4  IndexOptions=Index vector (dialog)  Indices=[1:2]  OutputSizes=1
  Selector1 : Selector  InputPortWidth=4  IndexOptions=Index vector (dialog)  Indices=[3:4]  OutputSizes=1
  Trigonometric Function : Trigonometry  Operator=atan
  Trigonometric Function1 : Trigonometry  Operator=atan
  alphalimit_hat : Outport  OutDataType=sfix(16)  OutScaling=2^0
  wires:
  muFz/1 -> Selector/1, Selector1/1
  Selector/1 -> MinMax/1
  MinMax/1 -> Gain/1
  Gain/1 -> Trigonometric Function/1
  Selector1/1 -> MinMax1/1
  MinMax1/1 -> Gain1/1
  Gain1/1 -> Trigonometric Function1/1
  Trigonometric Function/1 -> Mux/1
  Trigonometric Function1/1 -> Mux/2
  Mux/1 -> alphalimit_hat/1

== system debugECDD/Envelope control with Differential drive/envelope controller with DD/VSP_cal/prevent zero ==
  In1 : Inport  OutDataType=sfix(16)  OutScaling=2^0
  Abs : Abs
  Constant : Constant  Value=1/3.6  OutDataType=sfix(16)  OutScaling=2^0
  Product : Product  OutDataType=sfix(16)  OutScaling=2^0  RndMeth=Zero
  Relational Operator : RelationalOperator  Operator=>  LogicOutDataTypeMode=boolean  OutDataTypeStr=boolean
  Sign : Signum
  Switch : Switch  Threshold=0.5
  Switch1 : Switch  Threshold=0.5
  Unit Delay : UnitDelay  Orientation=left  X0=1  SampleTime=Ts
  Out1 : Outport  OutDataType=sfix(16)  OutScaling=2^0
  wires:
  Switch/1 -> Out1/1
  Relational Operator/1 -> Switch/2, Switch1/2
  Constant/1 -> Relational Operator/2, Product/1
  Abs/1 -> Relational Operator/1
  In1/1 -> Switch/1, Abs/1, Sign/1
  Sign/1 -> Switch1/1
  Product/1 -> Switch/3
  Switch1/1 -> Product/2, Unit Delay/1
  Unit Delay/1 -> Switch1/3

== system debugECDD/Envelope control with Differential drive/envelope controller with DD/target making/torque limit ==
  "drive trq " : Inport  OutDataType=sfix(16)  OutScaling=2^0
  Txlim drive : Inport  Port=2  OutDataType=sfix(16)  OutScaling=2^0
  MinMax4 : MinMax  Inputs=2  OutDataType=sfix(16)  OutScaling=2^0
  MinMax5 : MinMax  Function=max  Inputs=2  OutDataType=sfix(16)  OutScaling=2^0
  MinMax6 : MinMax  Inputs=2  OutDataType=sfix(16)  OutScaling=2^0
  MinMax7 : MinMax  Function=max  Inputs=2  OutDataType=sfix(16)  OutScaling=2^0
  Mux1 : Mux  Inputs=3
  Selector1 : Selector  InputPortWidth=4  IndexOptions=Index vector (dialog)  Indices=[1 2]  OutputSizes=1
  Selector10 : Selector  InputPortWidth=4  IndexOptions=Index vector (dialog)  Indices=1  OutputSizes=1
  Selector11 : Selector  InputPortWidth=4  IndexOptions=Index vector (dialog)  Indices=3  OutputSizes=1
  Selector12 : Selector  InputPortWidth=4  IndexOptions=Index vector (dialog)  Indices=2  OutputSizes=1
  Selector13 : Selector  InputPortWidth=4  IndexOptions=Index vector (dialog)  Indices=4  OutputSizes=1
  Selector8 : Selector  InputPortWidth=4  IndexOptions=Index vector (dialog)  Indices=3  OutputSizes=1
  Selector9 : Selector  InputPortWidth=4  IndexOptions=Index vector (dialog)  Indices=4  OutputSizes=1
  drive trq : Outport  OutDataType=sfix(16)  OutScaling=2^0
  wires:
  Selector8/1 -> MinMax4/1
  Selector10/1 -> MinMax4/2
  MinMax4/1 -> MinMax5/1
  Selector12/1 -> MinMax5/2
  Selector9/1 -> MinMax6/1
  Selector11/1 -> MinMax6/2
  MinMax6/1 -> MinMax7/1
  Selector13/1 -> MinMax7/2
  MinMax5/1 -> Mux1/2
  MinMax7/1 -> Mux1/3
  Mux1/1 -> drive trq/1
  "drive trq "/1 -> Selector9/1, Selector8/1, Selector1/1
  Txlim drive/1 -> Selector10/1, Selector12/1, Selector13/1, Selector11/1
  Selector1/1 -> Mux1/1

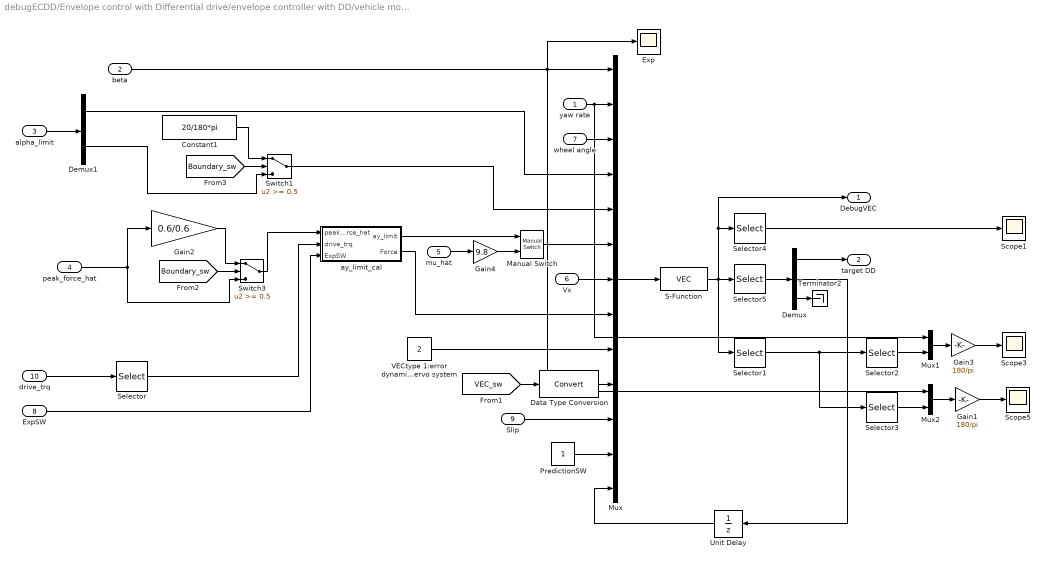
== system debugECDD/Envelope control with Differential drive/envelope controller with DD/vehicle motion control/EC ==
  yaw rate : Inport  OutDataType=sfix(16)  OutScaling=2^0
  beta : Inport  Port=2  OutDataType=sfix(16)  OutScaling=2^0
  alpha_limit : Inport  Port=3  OutDataType=sfix(16)  OutScaling=2^0
  peak_force_hat : Inport  Port=4  OutDataType=sfix(16)  OutScaling=2^0
  mu_hat : Inport  Port=5  OutDataType=sfix(16)  OutScaling=2^0
  Vx : Inport  Port=6  OutDataType=sfix(16)  OutScaling=2^0
  wheel angle : Inport  Port=7  OutDataType=sfix(16)  OutScaling=2^0
  ExpSW : Inport  Port=8  OutDataType=sfix(16)  OutScaling=2^0
  Slip : Inport  Port=9  OutDataType=sfix(16)  OutScaling=2^0
  drive_trq : Inport  Port=10  OutDataType=sfix(16)  OutScaling=2^0
  Constant1 : Constant  Value=20/180*pi  OutDataType=sfix(16)  OutScaling=2^0
  Data Type Conversion : DataTypeConversion  OutDataType=sfix(16)  OutScaling=2^0
  Demux : Demux  Outputs=[1 1 7]
  Demux1 : Demux  Outputs=2
  Exp : Scope
      settings: TimeRange=20  YMin=0  YMax=25  SaveName=ScopeData2
  Gain1 : Gain  Gain=180/pi  ParameterDataType=sfix(16)  ParameterScaling=2^0  OutDataType=sfix(16)  OutScaling=2^0
  Gain2 : Gain  Gain=0.6/0.6  ParameterDataType=sfix(16)  ParameterScaling=2^0  OutDataType=sfix(16)  OutScaling=2^0
  Gain3 : Gain  Gain=180/pi  ParameterDataType=sfix(16)  ParameterScaling=2^0  OutDataType=sfix(16)  OutScaling=2^0
  Gain4 : Gain  Gain=9.8  ParameterDataType=sfix(16)  ParameterScaling=2^0  OutDataType=sfix(16)  OutScaling=2^0
  Manual Switch : simulink/Signal Routing/Manual Switch  SystemSampleTime=-1  sw=0  action=0  varsize=off
  Mux : Mux  Inputs=13
  Mux1 : Mux  Inputs=2
  Mux2 : Mux  Inputs=2
  PredictionSW : Constant  OutDataType=sfix(16)  OutScaling=2^0
  S-Function : S-Function  FunctionName=VEC  Parameters=[a,b,c,q,K,Ks,0.01*100*Ku,Cfl,Crl,m,Iz]  EnableBusSupport=off
  Scope1 : Scope
      settings: TimeRange=20  YMin=0  YMax=25  SaveName=ScopeData3
  Scope3 : Scope
      settings: TimeRange=20  YMin=0  YMax=25  SaveName=ScopeData10
  Scope5 : Scope
      settings: YMin=-200  YMax=225  SaveName=ScopeData12
  Selector : Selector  InputPortWidth=4  IndexOptions=Index vector (dialog)  Indices=[3:4]  OutputSizes=1
  Selector1 : Selector  InputPortWidth=11  IndexOptions=Index vector (dialog)  Indices=[10;11]  OutputSizes=1
  Selector2 : Selector  InputPortWidth=2  IndexOptions=Index vector (dialog)  Indices=2  OutputSizes=1
  Selector3 : Selector  InputPortWidth=2  IndexOptions=Index vector (dialog)  Indices=1  OutputSizes=1
  Selector4 : Selector  InputPortWidth=11  IndexOptions=Index vector (dialog)  Indices=3  OutputSizes=1
  Selector5 : Selector  InputPortWidth=11  IndexOptions=Index vector (dialog)  Indices=[1:9]  OutputSizes=1
  Switch1 : Switch  Threshold=0.5
  Switch3 : Switch  Threshold=0.5
  Terminator2 : Terminator
  Unit Delay : UnitDelay  Orientation=left  SampleTime=0.002
  VECtype 1:error dynamics 2:servo system : Constant  Value=2  OutDataType=sfix(16)  OutScaling=2^0
  ay_limit_cal : Subsystem
  DebugVEC : Outport  OutDataType=sfix(16)  OutScaling=2^0
  target DD : Outport  Port=2  OutDataType=sfix(16)  OutScaling=2^0
  wires:
  [VEC_sw] -> Data Type Conversion/1
  Demux/3 -> Terminator2/1
  beta/1 -> Mux2/1, Mux/1, Exp/1
  S-Function/1 -> Selector5/1, Selector1/1, DebugVEC/1, Selector4/1
  Demux/2 -> Unit Delay/1
  Demux/1 -> target DD/1
  Mux/1 -> S-Function/1
  Vx/1 -> Mux/7
  wheel angle/1 -> Mux/3
  yaw rate/1 -> Mux/2, Mux1/1
  drive_trq/1 -> Selector/1
  Selector/1 -> ay_limit_cal/2(drive_trq)
  peak_force_hat/1 -> Gain2/1, Switch3/3
  Demux1/1 -> Mux/4
  alpha_limit/1 -> Demux1/1
  ExpSW/1 -> ay_limit_cal/3(ExpSW)
  Manual Switch/1 -> Mux/6
  ay_limit_cal/1(ay_limit) -> Manual Switch/1
  mu_hat/1 -> Gain4/1
  Data Type Conversion/1 -> Mux/10
  VECtype 1:error dynamics 2:servo system/1 -> Mux/9
  ay_limit_cal/2(Force) -> Mux/8
  Selector5/1 -> Demux/1
  Selector1/1 -> Selector2/1, Selector3/1
  Selector2/1 -> Mux1/2
  Mux1/1 -> Gain3/1
  Gain3/1 -> Scope3/1
  Selector3/1 -> Mux2/2
  Gain1/1 -> Scope5/1
  Mux2/1 -> Gain1/1
  Slip/1 -> Mux/11
  PredictionSW/1 -> Mux/12
  Unit Delay/1 -> Mux/13
  [Boundary_sw] -> Switch3/2
  Switch3/1 -> ay_limit_cal/1(peak_force_hat)
  Gain2/1 -> Switch3/1
  [Boundary_sw] -> Switch1/2
  Constant1/1 -> Switch1/1
  Switch1/1 -> Mux/5
  Demux1/2 -> Switch1/3
  Selector4/1 -> Scope1/1
  Gain4/1 -> Manual Switch/2

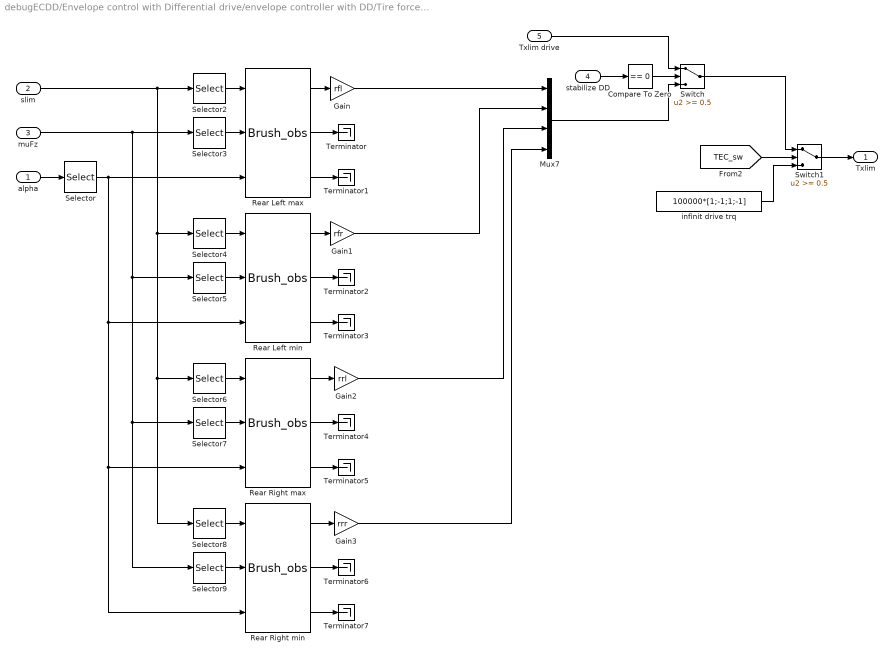
== system debugECDD/Envelope control with Differential drive/envelope controller with DD/Tire force control/limit_cal/Fx_limit_cal ==
  alpha : Inport  OutDataType=sfix(16)  OutScaling=2^0
  slim : Inport  Port=2  OutDataType=sfix(16)  OutScaling=2^0
  muFz : Inport  Port=3  OutDataType=sfix(16)  OutScaling=2^0
  stabilize DD : Inport  Port=4  OutDataType=sfix(16)  OutScaling=2^0
  Txlim drive : Inport  Port=5  OutDataType=sfix(16)  OutScaling=2^0
  Compare To Zero : simulink/Logic and Bit Operations/Compare To Zero  SystemSampleTime=-1  relop===  LogicOutDataTypeMode=uint8  ZeroCross=off
  Gain : Gain  Gain=rfl  ParameterDataType=sfix(16)  ParameterScaling=2^0  OutDataType=sfix(16)  OutScaling=2^0
  Gain1 : Gain  Gain=rfr  ParameterDataType=sfix(16)  ParameterScaling=2^0  OutDataType=sfix(16)  OutScaling=2^0
  Gain2 : Gain  Gain=rrl  ParameterDataType=sfix(16)  ParameterScaling=2^0  OutDataType=sfix(16)  OutScaling=2^0
  Gain3 : Gain  Gain=rrr  ParameterDataType=sfix(16)  ParameterScaling=2^0  OutDataType=sfix(16)  OutScaling=2^0
  Mux7 : Mux
  Rear Left max : S-Function  FunctionName=Brush_obs  Parameters=Crl, Crls, l  EnableBusSupport=off
  Rear Left min : S-Function  FunctionName=Brush_obs  Parameters=Crl, Crls, l  EnableBusSupport=off
  Rear Right max : S-Function  FunctionName=Brush_obs  Parameters=Crr, Crrs, l  EnableBusSupport=off
  Rear Right min : S-Function  FunctionName=Brush_obs  Parameters=Crr, Crrs, l  EnableBusSupport=off
  Selector : Selector  InputPortWidth=2  IndexOptions=Index vector (dialog)  Indices=2  OutputSizes=1
  Selector2 : Selector  InputPortWidth=4  IndexOptions=Index vector (dialog)  Indices=1  OutputSizes=1
  Selector3 : Selector  InputPortWidth=4  IndexOptions=Index vector (dialog)  Indices=3  OutputSizes=1
  Selector4 : Selector  InputPortWidth=4  IndexOptions=Index vector (dialog)  Indices=2  OutputSizes=1
  Selector5 : Selector  InputPortWidth=4  IndexOptions=Index vector (dialog)  Indices=3  OutputSizes=1
  Selector6 : Selector  InputPortWidth=4  IndexOptions=Index vector (dialog)  Indices=3  OutputSizes=1
  Selector7 : Selector  InputPortWidth=4  IndexOptions=Index vector (dialog)  Indices=4  OutputSizes=1
  Selector8 : Selector  InputPortWidth=4  IndexOptions=Index vector (dialog)  Indices=4  OutputSizes=1
  Selector9 : Selector  InputPortWidth=4  IndexOptions=Index vector (dialog)  Indices=4  OutputSizes=1
  Switch : Switch  Threshold=0.5  OutDataType=sfix(16)  OutScaling=2^0
  Switch1 : Switch  Threshold=0.5
  Terminator{,1..7} (8 alike) : Terminator
  infinit drive trq : Constant  Value=100000*[1;-1;1;-1]  OutDataType=sfix(16)  OutScaling=2^0
  Txlim : Outport  OutDataType=sfix(16)  OutScaling=2^0
  wires:
  Gain3/1 -> Mux7/4
  Gain1/1 -> Mux7/2
  Rear Right min/1 -> Gain3/1
  Rear Right max/1 -> Gain2/1
  Rear Left min/1 -> Gain1/1
  Rear Left max/1 -> Gain/1
  Rear Right min/3 -> Terminator7/1
  Rear Right min/2 -> Terminator6/1
  Rear Right max/3 -> Terminator5/1
  Rear Right max/2 -> Terminator4/1
  Rear Left min/3 -> Terminator3/1
  Rear Left min/2 -> Terminator2/1
  Rear Left max/3 -> Terminator1/1
  Rear Left max/2 -> Terminator/1
  Selector/1 -> Rear Right max/3, Rear Right min/3, Rear Left min/3, Rear Left max/3
  muFz/1 -> Selector7/1, Selector9/1, Selector5/1, Selector3/1
  slim/1 -> Selector6/1, Selector8/1, Selector4/1, Selector2/1
  Selector9/1 -> Rear Right min/2
  Selector8/1 -> Rear Right min/1
  Selector7/1 -> Rear Right max/2
  Selector6/1 -> Rear Right max/1
  Selector5/1 -> Rear Left min/2
  Selector4/1 -> Rear Left min/1
  Selector3/1 -> Rear Left max/2
  Selector2/1 -> Rear Left max/1
  alpha/1 -> Selector/1
  Gain/1 -> Mux7/1
  Gain2/1 -> Mux7/3
  [TEC_sw] -> Switch1/2
  Switch1/1 -> Txlim/1
  infinit drive trq/1 -> Switch1/3
  Compare To Zero/1 -> Switch/2
  stabilize DD/1 -> Compare To Zero/1
  Mux7/1 -> Switch/3
  Txlim drive/1 -> Switch/1
  Switch/1 -> Switch1/1

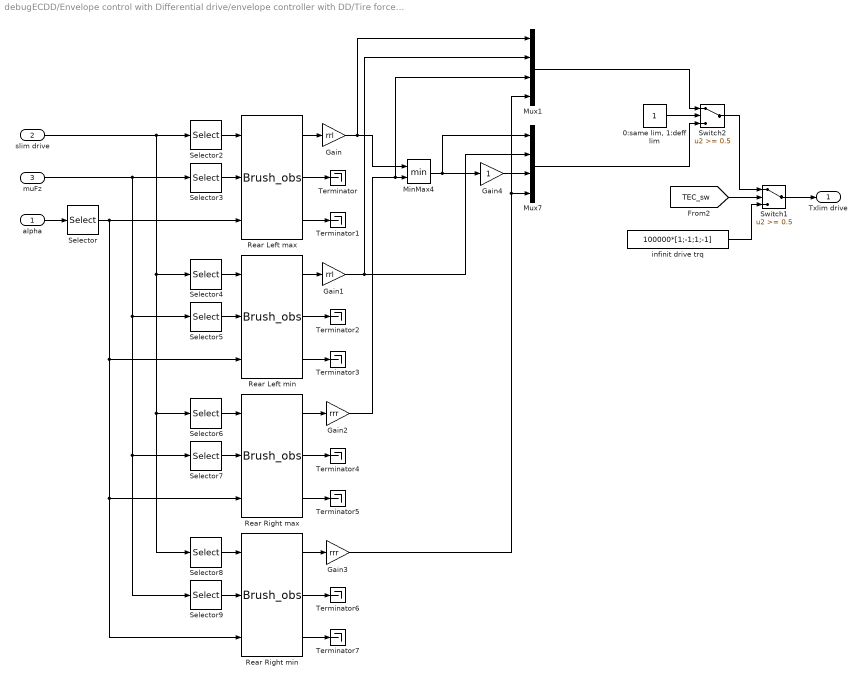
== system debugECDD/Envelope control with Differential drive/envelope controller with DD/Tire force control/limit_cal/Fx_limit_cal1 ==
  alpha : Inport  OutDataType=sfix(16)  OutScaling=2^0
  slim drive : Inport  Port=2  OutDataType=sfix(16)  OutScaling=2^0
  muFz : Inport  Port=3  OutDataType=sfix(16)  OutScaling=2^0
  "0:same lim, 1:deff lim" : Constant  OutDataType=sfix(16)  OutScaling=2^0
  Gain : Gain  Gain=rrl  ParameterDataType=sfix(16)  ParameterScaling=2^0  OutDataType=sfix(16)  OutScaling=2^0
  Gain1 : Gain  Gain=rrl  ParameterDataType=sfix(16)  ParameterScaling=2^0  OutDataType=sfix(16)  OutScaling=2^0
  Gain2 : Gain  Gain=rrr  ParameterDataType=sfix(16)  ParameterScaling=2^0  OutDataType=sfix(16)  OutScaling=2^0
  Gain3 : Gain  Gain=rrr  ParameterDataType=sfix(16)  ParameterScaling=2^0  OutDataType=sfix(16)  OutScaling=2^0
  Gain4 : Gain  ParameterDataType=sfix(16)  ParameterScaling=2^0  OutDataType=sfix(16)  OutScaling=2^0
  MinMax4 : MinMax  Inputs=2  OutDataType=sfix(16)  OutScaling=2^0
  Mux1 : Mux
  Mux7 : Mux
  Rear Left max : S-Function  FunctionName=Brush_obs  Parameters=Crl, Crls, l  EnableBusSupport=off
  Rear Left min : S-Function  FunctionName=Brush_obs  Parameters=Crl, Crls, l  EnableBusSupport=off
  Rear Right max : S-Function  FunctionName=Brush_obs  Parameters=Crr, Crrs, l  EnableBusSupport=off
  Rear Right min : S-Function  FunctionName=Brush_obs  Parameters=Crr, Crrs, l  EnableBusSupport=off
  Selector : Selector  InputPortWidth=2  IndexOptions=Index vector (dialog)  Indices=2  OutputSizes=1
  Selector2 : Selector  InputPortWidth=4  IndexOptions=Index vector (dialog)  Indices=1  OutputSizes=1
  Selector3 : Selector  InputPortWidth=4  IndexOptions=Index vector (dialog)  Indices=3  OutputSizes=1
  Selector4 : Selector  InputPortWidth=4  IndexOptions=Index vector (dialog)  Indices=2  OutputSizes=1
  Selector5 : Selector  InputPortWidth=4  IndexOptions=Index vector (dialog)  Indices=3  OutputSizes=1
  Selector6 : Selector  InputPortWidth=4  IndexOptions=Index vector (dialog)  Indices=3  OutputSizes=1
  Selector7 : Selector  InputPortWidth=4  IndexOptions=Index vector (dialog)  Indices=4  OutputSizes=1
  Selector8 : Selector  InputPortWidth=4  IndexOptions=Index vector (dialog)  Indices=4  OutputSizes=1
  Selector9 : Selector  InputPortWidth=4  IndexOptions=Index vector (dialog)  Indices=4  OutputSizes=1
  Switch1 : Switch  Threshold=0.5
  Switch2 : Switch  Threshold=0.5
  Terminator{,1..7} (8 alike) : Terminator
  infinit drive trq : Constant  Value=100000*[1;-1;1;-1]  OutDataType=sfix(16)  OutScaling=2^0
  Txlim drive : Outport  OutDataType=sfix(16)  OutScaling=2^0
  wires:
  Gain2/1 -> MinMax4/2, Mux1/3
  alpha/1 -> Selector/1
  Selector2/1 -> Rear Left max/1
  Selector3/1 -> Rear Left max/2
  Selector4/1 -> Rear Left min/1
  Selector5/1 -> Rear Left min/2
  Selector6/1 -> Rear Right max/1
  Selector7/1 -> Rear Right max/2
  Selector8/1 -> Rear Right min/1
  Selector9/1 -> Rear Right min/2
  slim drive/1 -> Selector2/1, Selector4/1, Selector8/1, Selector6/1
  muFz/1 -> Selector3/1, Selector5/1, Selector9/1, Selector7/1
  Selector/1 -> Rear Left max/3, Rear Left min/3, Rear Right min/3, Rear Right max/3
  Rear Left max/2 -> Terminator/1
  Rear Left max/3 -> Terminator1/1
  Rear Left min/2 -> Terminator2/1
  Rear Left min/3 -> Terminator3/1
  Rear Right max/2 -> Terminator4/1
  Rear Right max/3 -> Terminator5/1
  Rear Right min/2 -> Terminator6/1
  Rear Right min/3 -> Terminator7/1
  Rear Left max/1 -> Gain/1
  Rear Left min/1 -> Gain1/1
  Rear Right max/1 -> Gain2/1
  Rear Right min/1 -> Gain3/1
  Gain1/1 -> Mux7/2, Mux1/2
  Gain3/1 -> Mux7/4, Mux1/4
  [TEC_sw] -> Switch1/2
  infinit drive trq/1 -> Switch1/3
  Switch1/1 -> Txlim drive/1
  MinMax4/1 -> Mux7/1, Gain4/1
  Gain/1 -> MinMax4/1, Mux1/1
  Gain4/1 -> Mux7/3
  Mux7/1 -> Switch2/3
  Mux1/1 -> Switch2/1
  Switch2/1 -> Switch1/1
  "0:same lim, 1:deff lim"/1 -> Switch2/2
